simulink model "simplified_sim1"  (R2018b)
settings: Solver=FixedStepAuto  StartTime=0.0  StopTime=400  FixedStep=fswParams.sample_time_s  RelTol=1e-3
libraries: MEKF_Inputs_lib x2, Environment_lib x1, MEKF_lib x1, Sensors_Lib x1, satelliteDynamics_lib x1
settings Model: Creator=satcave1  LastModifiedBy=kylle

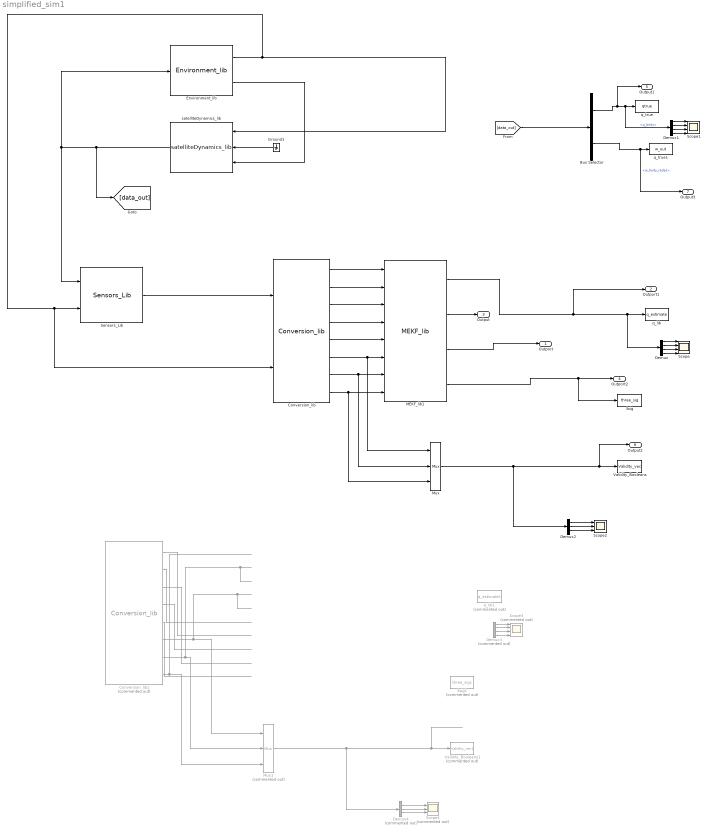
== system simplified_sim1 ==
  3sig : ToWorkspace  VariableName=three_sig  SaveFormat=Timeseries  SampleTime=-1
  3sig1 : ToWorkspace  Commented=on  VariableName=three_sig1  SaveFormat=Timeseries  SampleTime=-1
  Bus Selector : BusSelector  OutputSignals=q_body,w_body_radps
  Conversion_lib : MEKF_Inputs_lib/Conversion_lib  SystemSampleTime=-1
  Conversion_lib1 : MEKF_Inputs_lib/Conversion_lib  Commented=on  SystemSampleTime=-1
  Demux : Demux
  Demux1 : Demux
  Demux2 : Demux  Outputs=3
  Demux3 : Demux  Commented=on
  Demux4 : Demux  Commented=on  Outputs=3
  Environment_lib : Environment_lib/Environment_lib  SystemSampleTime=-1
  Ground1 : Ground
  MEKF_lib1 : MEKF_lib/MEKF_lib  SystemSampleTime=-1
  Mux : Mux  Inputs=3
  Mux1 : Mux  Commented=on  Inputs=3
  Scope : Scope  NumInputPorts=4
  Scope1 : Scope  NumInputPorts=4
  Scope2 : Scope  NumInputPorts=3
  Scope3 : Scope  Commented=on  NumInputPorts=4
  Scope4 : Scope  Commented=on  NumInputPorts=3
  Sensors_Lib : Sensors_Lib/Sensors_Lib  SystemSampleTime=-1
  Validity_Booleans : ToWorkspace  VariableName=Validity_vec  SaveFormat=Timeseries  SampleTime=-1
  Validity_Booleans1 : ToWorkspace  Commented=on  VariableName=Validity_vec1  SaveFormat=Timeseries  SampleTime=-1
  q_lib : ToWorkspace  VariableName=q_estimate  SaveFormat=Timeseries  SampleTime=-1
  q_lib1 : ToWorkspace  Commented=on  VariableName=q_estimate1  SaveFormat=Timeseries  SampleTime=-1
  q_true : ToWorkspace  VariableName=qtrue  SaveFormat=Timeseries  SampleTime=-1
  q_true1 : ToWorkspace  VariableName=w_out  SaveFormat=Timeseries  SampleTime=-1
  satelliteDynamics_lib : satelliteDynamics_lib/satelliteDynamics_lib  SystemSampleTime=-1
  Outport : Outport
  Outport1 : Outport  Port=2
  Output : Outport  Port=3
  Outport2 : Outport  Port=4
  Output1 : Outport  Port=5
  Output2 : Outport  Port=6
  Output3 : Outport  Port=7
  wires:
  satelliteDynamics_lib/1 -> [data_out], Environment_lib/1, Sensors_Lib/1
  Ground1/1 -> satelliteDynamics_lib/2
  Environment_lib/2 -> satelliteDynamics_lib/3
  [data_out] -> Bus Selector/1
  Bus Selector/1 -> Output1/1, Demux1/1, q_true/1  "<q_body>"
  Bus Selector/2 -> Output3/1, q_true1/1  "<w_body_radps>"
  Environment_lib/1 -> Conversion_lib/2, Sensors_Lib/2, satelliteDynamics_lib/1
  Conversion_lib/6 -> MEKF_lib1/6, Mux/1
  Conversion_lib/7 -> MEKF_lib1/7, Mux/2
  Conversion_lib/8 -> MEKF_lib1/8, Mux/3
  Sensors_Lib/1 -> Conversion_lib/1
  Demux/1 -> Scope/1
  Demux/2 -> Scope/2
  Demux/3 -> Scope/3
  Demux/4 -> Scope/4
  Demux1/3 -> Scope1/3
  Demux1/2 -> Scope1/2
  Demux1/4 -> Scope1/4
  Demux1/1 -> Scope1/1
  Demux2/3 -> Scope2/3
  Demux2/2 -> Scope2/2
  Mux/1 -> Demux2/1, Output2/1, Validity_Booleans/1
  Demux2/1 -> Scope2/1
  ? -> ?
  Conversion_lib1/3 -> ?
  Demux3/4 -> Scope3/4
  Demux3/2 -> Scope3/2
  ? -> 3sig1/1
  ? -> q_lib1/1
  Conversion_lib1/1 -> ?
  Conversion_lib1/2 -> ?
  ? -> ?
  Conversion_lib1/5 -> ?
  Conversion_lib1/4 -> ?
  Demux4/2 -> Scope4/2
  Demux4/1 -> Scope4/1
  Mux1/1 -> Demux4/1, Validity_Booleans1/1
  Conversion_lib1/8 -> Mux1/3
  Conversion_lib1/6 -> Mux1/1
  Demux4/3 -> Scope4/3
  Demux3/1 -> Scope3/1
  Conversion_lib1/7 -> Mux1/2
  Demux3/3 -> Scope3/3
  Conversion_lib/1 -> MEKF_lib1/1
  Conversion_lib/2 -> MEKF_lib1/2
  Conversion_lib/3 -> MEKF_lib1/3
  Conversion_lib/4 -> MEKF_lib1/4
  Conversion_lib/5 -> MEKF_lib1/5
  MEKF_lib1/2 -> Output/1
  MEKF_lib1/1 -> Demux/1, q_lib/1, Outport1/1
  MEKF_lib1/3 -> Outport/1
  MEKF_lib1/4 -> 3sig/1, Outport2/1
